simulink model "sim2020_7_21_v2"  (R2017a)
settings: Solver=ode45  StartTime=0.0  StopTime=20  FixedStep=0.0001  MaxStep=0.05  MinStep=0.04  RelTol=1e-3
libraries: simulink x1
settings Model: Creator=asus  LastModifiedBy=Lenovo

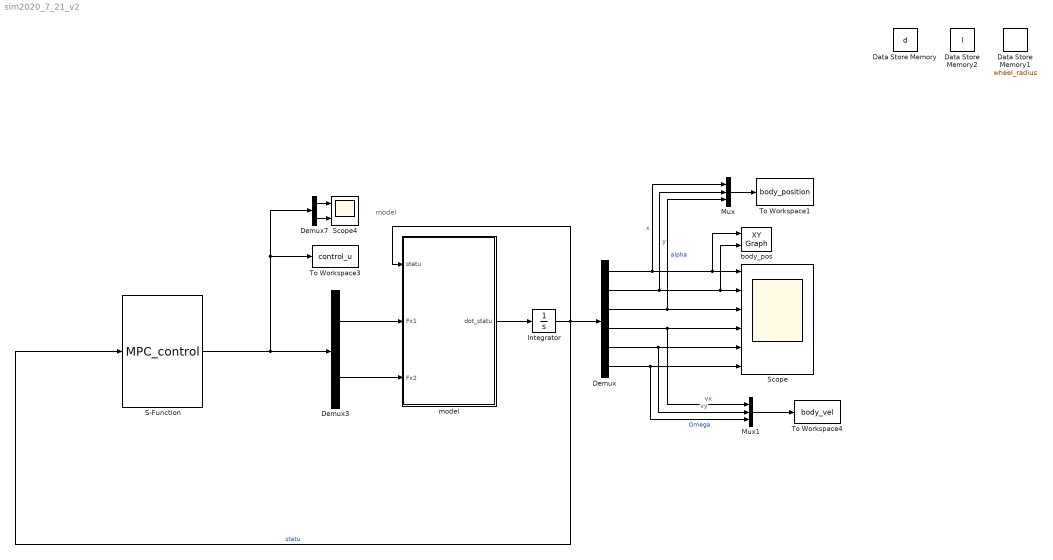
== system sim2020_7_21_v2 ==
  note: model
  Data Store Memory : DataStoreMemory  DataStoreName=d  ReadBeforeWriteMsg=warning  WriteAfterWriteMsg=warning  WriteAfterReadMsg=warning  ShowAdditionalParam=off  OutDataTypeStr=double
  Data Store Memory1 : DataStoreMemory  DataStoreName=wheel_radius  ReadBeforeWriteMsg=warning  WriteAfterWriteMsg=warning  WriteAfterReadMsg=warning  ShowAdditionalParam=off  OutDataTypeStr=double
  Data Store Memory2 : DataStoreMemory  DataStoreName=l  ReadBeforeWriteMsg=warning  WriteAfterWriteMsg=warning  WriteAfterReadMsg=warning  ShowAdditionalParam=off  OutDataTypeStr=double
  Demux : Demux  Outputs=6
  Demux3 : Demux  Outputs=2
  Demux7 : Demux  Outputs=2
  Integrator : Integrator  InitialCondition=[2 -2 pi/2 0 0 0]  IgnoreLimit=on
  Mux : Mux  Inputs=3
  Mux1 : Mux  Inputs=3
  S-Function : S-Function  FunctionName=MPC_control  SFunctionDeploymentMode=off  EnableBusSupport=off
  Scope : Scope  NumInputPorts=6
  Scope4 : Scope  NumInputPorts=2
  To Workspace1 : ToWorkspace  VariableName=body_position  SampleTime=-1
  To Workspace3 : ToWorkspace  VariableName=control_u  SampleTime=-1
  To Workspace4 : ToWorkspace  VariableName=body_vel  SampleTime=-1
  body_pos : simulink/Sinks/XY Graph  xmin=-10  xmax=10  ymin=-10  ymax=10  st=-1
  model : MATLAB Function  TreatAsAtomicUnit=on
  wires:
  Integrator/1 -> S-Function/1, model/1(statu), Demux/1  "statu"
  Demux/3 -> Mux/3, Scope/3  "alpha"
  Demux/1 -> Mux/1, body_pos/1, Scope/1  "x"
  Demux/2 -> Mux/2, body_pos/2, Scope/2  "y"
  Demux7/2 -> Scope4/2
  Demux7/1 -> Scope4/1
  model/1(dot_statu) -> Integrator/1
  Demux/4 -> Mux1/1, Scope/4  "vx"
  Demux/5 -> Mux1/2, Scope/5  "vy"
  Demux/6 -> Mux1/3, Scope/6  "Omega"
  Demux3/1 -> model/2(Fx1)
  Demux3/2 -> model/3(Fx2)
  Mux1/1 -> To Workspace4/1
  Mux/1 -> To Workspace1/1
  S-Function/1 -> Demux3/1, To Workspace3/1, Demux7/1

== matlab function sim2020_7_21_v2/model ==
  data: statu input; dot_statu output; wheel_radius data_store_memory; l data_store_memory; d data_store_memory; Fx1 input; Fx2 input
function dot_statu = model(statu, Fx1 , Fx2 )
global wheel_radius d l ;
wheel_radius = 0.330/2;
d = 0.18;
l = 0.16;
m = 24;
Iz = 11.89;
c = 513.6; %轮胎侧偏刚度


x = statu(1);
y = statu(2);
alpha = statu(3);
vx = statu(4);
vy = statu(5);
omega = statu(6);

dot_x = vx*cos(alpha)-vy*sin(alpha);
dot_y = vx*sin(alpha)+vy*cos(alpha);
dot_alpha = omega;
dot_vx = (Fx1+Fx2)/m;
dot_vy = (-2*c*(vy+l*omega))/(m*vx);
dot_omega = (Fx2-Fx1)*d/(Iz)+(2*c*l*(vy+l*omega))/(Iz*vx);

% 状态【x y alpha vx vy omega】
dot_statu = [dot_x; dot_y; dot_alpha; dot_vx; dot_vy; dot_omega]; 

end

% max=1/wheel_radius;
% for i=1:size(wheel_omega,2)
%     if wheel_omega(i)>max
%         wheel_omega(i) = max;
%     else
%         if wheel_omega(i)<-max
%             wheel_omega(i) = -max;
%         else
%             wheel_omega(i) = wheel_omega(i);
%         end
%     end
% end
